simulink library "cstblocks"  (R2025b)
settings: Solver=ode45  StartTime=0.0  StopTime=10.0  RelTol=1e-3
values from neighbouring files (symbols this model uses):
  D = ltipack.lftdataFRD(IC,ltipack.LFTBlockWrapper(blk))    [ControlDesignBlock.m]    (also in DynamicBlock.m = pidstd(ltipack_ssdata(blk)); delayss.m = ltipack.ssdata(a0,b,c,[d0 q;s zeros(length(tau))],[],Ts))
  Ts = blk.Ts_    [DynamicBlock.m]    (also in delayss.m = varargin{1})
undefined symbols (not defined in the file or in its folder): AA, BB, CC, DD, Discrete, INFO, rss, set, Time, uDelay, V, xinit, yDelay
libraries: $bdroot x4, slpidlib x4, cstextras x4, sharedTrackingLibrary x3, ctrlSharedLib x1
(part 2 of 3)

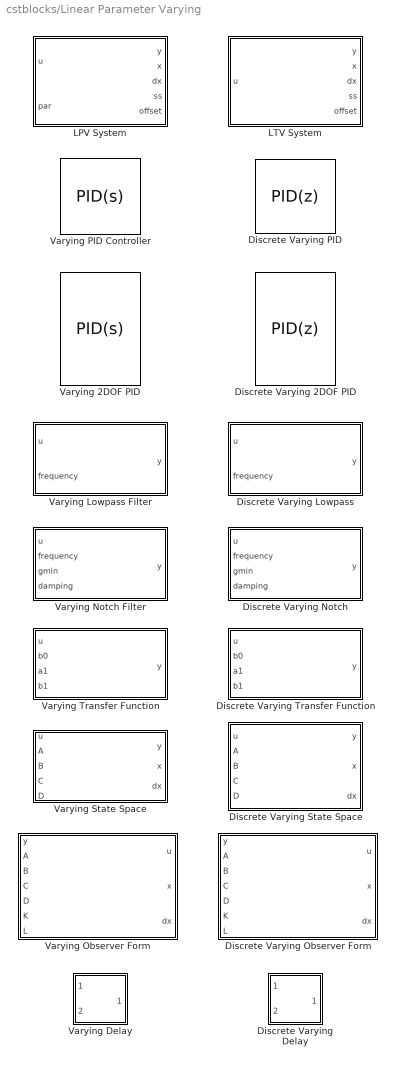
== system cstblocks/Linear Parameter Varying ==
  Discrete Varying 2DOF PID : slpidlib/PID Controller (2DOF)  Controller=PID  Form=Parallel  TimeDomain=Discrete-time  UseExternalTs=off  SampleTime=-1  IntegratorMethod=Forward Euler  FilterMethod=Forward Euler  ControllerParametersSource=external  P=1  I=1  UseKiTs=off  D=0  UseExternalDerivativeSource=off  N=100  UseFilter=on  b=1  c=1  TunerSelectOption=Transfer Function Based (PID Tuner App)  InitialConditionSource=internal  InitialConditionForIntegrator=0  InitialConditionForFilter=0  DifferentiatorICPrevScaledInput=0  ExternalReset=none  TrackingMode=off  Kt=1  LimitOutput=off  SatLimitsSource=internal  UpperSaturationLimit=inf  LowerSaturationLimit=-inf  LinearizeAsGain=on  AntiWindupMode=none  Kb=1  LimitIntegrator=off  UpperIntegratorSaturationLimit=inf  LowerIntegratorSaturationLimit=-inf  POutMin=[]  POutMax=[]  IOutMin=[]  IOutMax=[]  DOutMin=[]  DOutMax=[]  NOutMin=[]  NOutMax=[]  bOutMin=[]  bOutMax=[]  cOutMin=[]  cOutMax=[]  SumOutMin=[]  SumOutMax=[]  SaturationOutMin=[]  SaturationOutMax=[]  PParamMin=[]  PParamMax=[]  IParamMin=[]  IParamMax=[]  DParamMin=[]  DParamMax=[]  NParamMin=[]  NParamMax=[]  bParamMin=[]  bParamMax=[]  cParamMin=[]  cParamMax=[]  KbParamMin=[]  KbParamMax=[]  KtParamMin=[]  KtParamMax=[]  KbOutMin=[]  KbOutMax=[]  KtOutMin=[]  KtOutMax=[]  IntegratorOutMin=[]  IntegratorOutMax=[]  FilterOutMin=[]  FilterOutMax=[]  SumI1OutMin=[]  SumI1OutMax=[]  SumI2OutMin=[]  SumI2OutMax=[]  SumI3OutMin=[]  SumI3OutMax=[]  SumI4OutMin=[]  SumI4OutMax=[]  SumDOutMin=[]  SumDOutMax=[]  Sum1OutMin=[]  Sum1OutMax=[]  Sum2OutMin=[]  Sum2OutMax=[]  Sum3OutMin=[]  Sum3OutMax=[]  DifferentiatorOutMin=[]  DifferentiatorOutMax=[]  FilterDiffOutCoefMin=[]  FilterDiffOutCoefMax=[]  ReciprocalOutMin=[]  ReciprocalOutMax=[]  SumDenOutMin=[]  SumDenOutMax=[]  SumNumOutMin=[]  SumNumOutMax=[]  DivideOutMin=[]  DivideOutMax=[]  UdiffTsProdOutMin=[]  UdiffTsProdOutMax=[]  NTsProdOutMin=[]  NTsProdOutMax=[]  UintegralTsProdOutMin=[]  UintegralTsProdOutMax=[]  UngainTsProdOutMin=[]  UngainTsProdOutMax=[]  ClampingZeroOutDataTypeStr=Inherit: Inherit via back propagation  ClampingZeroOutMin=[]  ClampingZeroOutMax=[]  FilterDenConstantOutDataTypeStr=Inherit: Inherit via back propagation  FilterDenConstantOutMin=[]  FilterDenConstantOutMax=[]  PCopyOutDataTypeStr=Inherit: Inherit via back propagation  PCopyOutMin=[]  PCopyOutMax=[]  NCopyOutDataTypeStr=Inherit: Inherit via back propagation  NCopyOutMin=[]  NCopyOutMax=[]  IntegratorContinuousStateAttributes=''  IntegratorStateMustResolveToSignalObject=off  IntegratorRTWStateStorageClass=Auto  FilterContinuousStateAttributes=''  FilterStateMustResolveToSignalObject=off  FilterRTWStateStorageClass=Auto  ParallelPVariant=ExternalParameters  IdealPVariant=Disabled  IVariant=ExternalParameters  DVariant=ExternalParameters  bVariant=ExternalParameters  cVariant=ExternalParameters  IntegratorVariant=Discrete  SatVariant=Disabled  AWVariant=Passthrough  PCopyVariant=Disabled  TRVariant=Disabled  FdbkBlocksVariant=Forward  IdealPFdbkVariant=Disabled  SatFdbkVariant=Disabled  DerivativeFilterVariant=ForwardEulerFilter  NVariant=ExternalParameters  NCopyVariant=Disabled  FilterICVariant=InternalICsFilter  IntegratorICVariant=InternalICs  ExternalResetVariant=Disabled  TRSumVariant=Passthrough  SumFdbkVariant=Disabled  SumVariant=Sum_PID  TsampFilterVariant=InternalTs  TsampNgainVariant=Passthrough  TsampIntegralVariant=Disabled_SignalSpec  ExternalSaturationOutDataTypeStr=Inherit: Same as second input  DerivativeSourceVariant=ErrorSignal  PreIntVariant=InternalPreInt
  Discrete Varying Delay : Subsystem  mask(Discrete Varying Delay){Td=1, TdMax=10, TdFixed=[], u0=0, Ts=-1, PreventDirectFeedthrough=off}
      mask prompts: Td "Control:simulink:VaryingDelayLabel8"; TdMax "Control:simulink:VaryingDelayLabel2"; TdFixed "Control:simulink:VaryingDelayLabel4"; u0 "Control:simulink:VaryingDelayLabel5"; Ts "Control:simulink:VaryingSSLabel5"; PreventDirectFeedthrough "Control:simulink:VaryingDelayLabel9"
      mask help: Control:simulink:VaryingDelay3
      mask init:
      | df = get_param(bdroot,'dirty');
      | if ~(Ts>0 || Ts==-1)
      |    DAStudio.slerror('Control:simulink:InvalidTs',get_param(gcb,'handle'))
      | end
      | n = max([numel(Td) numel(TdMax) numel(u0)]);
      | if isscalar(Td), Td = repmat(Td,[1 n]); end
      | if isscalar(TdMax), TdMax = repmat(TdMax,[1 n]); end
      | if isscalar(u0), u0 = repmat(u0,[1 n]); end
      | if ~isequal(numel(Td),numel(TdMax),numel(u0))
      |    DAStudio.slerror('Control:simulink:VaryingDelay1',get_param(gcb,'handle'))
      | elseif any(TdFixed>n)
      |    DAStudio.slerror('Control:simulink:VaryingDelay4',get_param(gcb,'handle'))
      | end
      | 
      | % Build representation of delay vector
      | Options = struct('PreventDirectFeedthrough',PreventDirectFeedthrough);
      | controllib.internal.blocks.varying.varyingDelay(gcb,Ts,Td,TdFixed,Options);
      | set_param(bdroot,'dirty',df)
      mask Help: eval('helpview("control","DiscreteVaryingDelayBlock");')
      mask DialogControl Td Prompt: Nominal delay (number of samples):
      mask DialogControl TdMax Prompt: Maximum delay:
      mask DialogControl TdFixed Prompt: Fixed delays (indices):
      mask DialogControl u0 Prompt: Initial output:
      mask DialogControl Ts Prompt: Sample time (-1 for inherited):
      mask DialogControl PreventDirectFeedthrough Prompt: Prevent direct feedthrough with minimum delay of 1
      mask Display: block_icon('Delay')
  Discrete Varying Lowpass : Subsystem  mask(Discrete Varying Lowpass){N=1, w0=0, Ts=1}
      mask prompts: N "Control:simulink:VaryingLowpassLabel1"; w0 "Control:simulink:VaryingLowpassLabel2"; Ts "Control:simulink:VaryingLowpassLabel3"
      mask help: Control:simulink:VaryingLowpass2
      mask init:
      | if N~=round(N)
      |    hCB = get_param(gcb,'handle');
      |    DAStudio.slerror('Control:simulink:InvalidOrder',hCB)
      | elseif w0*Ts>=pi
      |    hCB = get_param(gcb,'handle');
      |    DAStudio.slerror('Control:simulink:InvalidPrewarp',hCB)
      | end
      | SimStatus = get_param(bdroot,'SimulationStatus');
      | if any(strcmp(SimStatus,{'initializing','updating','stopped'}))
      |    controllib.internal.blocks.varying.varyingLP(gcb,N,Ts)
      | end
      mask Help: eval('helpview(''control'',''VaryingLowpassDT'');')
      mask DialogControl N Prompt: Filter order:
      mask DialogControl w0 Prompt: Pre-warping frequency w0 (rad/s):
      mask DialogControl Ts Prompt: Sample time Ts:
      mask Display:
      | image('lowpass_dt.png',[0.1 0 0.8 1]);
      | port_label('input', 2, 'freq');
  Discrete Varying Notch : Subsystem  mask(Discrete Varying Notch){w0=0, Ts=1}
      mask prompts: w0 "Control:simulink:VaryingLowpassLabel2"; Ts "Control:simulink:VaryingLowpassLabel3"
      mask help: Control:simulink:VaryingNotch2
      mask init:
      | if w0*Ts>=pi
      |    hCB = get_param(gcb,'handle');
      |    DAStudio.slerror('Control:simulink:InvalidPrewarp',hCB)
      | elseif w0>0
      |    tau = tan(w0*Ts/2)/w0;
      | else
      |    tau = Ts/2;
      | end
      mask Help: eval('helpview(''control'',''VaryingNotchDT'');')
      mask DialogControl w0 Prompt: Pre-warping frequency w0 (rad/s):
      mask DialogControl Ts Prompt: Sample time Ts:
      mask Display:
      | image('notch_dt.png',[0.1 0 0.8 1])
      | port_label('input', 2, 'freq')
      | port_label('input', 3, 'gmin')
      | port_label('input', 4, 'damp')
  Discrete Varying Observer Form : Subsystem  mask(Discrete Varying Observer Form){x0=0, Ts=-1, OutputX=on, OutputDX=on}
      mask prompts: x0 "Control:simulink:VaryingSSLabel1"; Ts "Control:simulink:VaryingSSLabel5"; OutputX "Control:simulink:VaryingSSLabel3"; OutputDX "Control:simulink:VaryingSSLabel4"
      mask help: Control:simulink:VaryingObserver2
      mask init:
      | % Use exact linearization of product block
      | % pblks = find_system(gcb,'FollowLinks','on',...
      | %    'LookUnderMasks','all','SearchDepth',1,'BlockType','Product');
      | % rep = struct(...
      | %    'Specification','controllib.internal.blocks.matrixProductJacobian',...
      | %    'Type','Function',...
      | %    'ParameterNames','',...
      | %    'ParameterValues','');
      | % for i=1:numel(pblks)
      | %    set_param(pblks{i},...
      | %       'SCDEnableBlockLinearizationSpecification','on',...
      | %       'SCDBlockLinearizationSpecification',rep)
      | % end
      | SimStatus = get_param(bdroot,'SimulationStatus');
      | if any(strcmp(SimStatus,{'initializing','updating','stopped'}))
      |    controllib.internal.blocks.varying.varyingOF(gcb,OutputX,OutputDX);
      | end
      mask Help: eval('helpview(''control'',''VaryingObserverDT'');')
      mask DialogControl Ts Prompt: Sample time (-1 for inherited):
      mask DialogControl OutputX Prompt: Output states
      mask DialogControl OutputDX Prompt: Output state derivatives
      mask Display:
      | port_label('input', 1, 'y_k','texmode','on')
      | port_label('input', 2, 'A')
      | port_label('input', 3, 'B')
      | port_label('input', 4, 'C')
      | port_label('input', 5, 'D')
      | port_label('input', 6, 'K')
      | port_label('input', 7, 'L')
      | port_label('output', 1, 'u_k','texmode','on')
      | next_ = 2;
      | if OutputX
      |    port_label('output', next_, 'x_k','texmode','on')
      |    next_ = next_+1;
      | end
      | if OutputDX
      |    port_label('output', next_, 'x_{k+1}','texmode','on')
      |    next_ = next_+1;
      | end
      | text(0.5,0.7,'x_{k+1} = A x_k + B u_k + L \epsilon_k',...
      |    'horizontalAlignment', 'center','texmode','on')
      | text(0.5,0.5,'u_k = -K x_k',...
      |    'horizontalAlignment', 'center','texmode','on')
      | text(0.5,0.3,'\epsilon_k = y_k - C x_k - D u_k',...
      |    'horizontalAlignment', 'center','texmode','on')
  Discrete Varying PID : slpidlib/PID Controller  Controller=PID  Form=Parallel  TimeDomain=Discrete-time  UseExternalTs=off  SampleTime=-1  IntegratorMethod=Forward Euler  FilterMethod=Forward Euler  ControllerParametersSource=external  P=1  I=1  UseKiTs=off  D=0  UseExternalDerivativeSource=off  N=100  UseFilter=on  TunerSelectOption=Transfer Function Based (PID Tuner App)  InitialConditionSource=internal  InitialConditionForIntegrator=0  InitialConditionForFilter=0  DifferentiatorICPrevScaledInput=0  ExternalReset=none  TrackingMode=off  Kt=1  LimitOutput=off  SatLimitsSource=internal  UpperSaturationLimit=inf  LowerSaturationLimit=-inf  LinearizeAsGain=on  AntiWindupMode=none  Kb=1  LimitIntegrator=off  UpperIntegratorSaturationLimit=inf  LowerIntegratorSaturationLimit=-inf  POutMin=[]  POutMax=[]  IOutMin=[]  IOutMax=[]  DOutMin=[]  DOutMax=[]  NOutMin=[]  NOutMax=[]  SumOutMin=[]  SumOutMax=[]  SaturationOutMin=[]  SaturationOutMax=[]  PParamMin=[]  PParamMax=[]  IParamMin=[]  IParamMax=[]  DParamMin=[]  DParamMax=[]  NParamMin=[]  NParamMax=[]  KbParamMin=[]  KbParamMax=[]  KtParamMin=[]  KtParamMax=[]  KbOutMin=[]  KbOutMax=[]  KtOutMin=[]  KtOutMax=[]  IntegratorOutMin=[]  IntegratorOutMax=[]  FilterOutMin=[]  FilterOutMax=[]  SumI1OutMin=[]  SumI1OutMax=[]  SumI2OutMin=[]  SumI2OutMax=[]  SumI3OutMin=[]  SumI3OutMax=[]  SumI4OutMin=[]  SumI4OutMax=[]  SumDOutMin=[]  SumDOutMax=[]  DifferentiatorOutMin=[]  DifferentiatorOutMax=[]  FilterDiffOutCoefMin=[]  FilterDiffOutCoefMax=[]  ReciprocalOutMin=[]  ReciprocalOutMax=[]  SumDenOutMin=[]  SumDenOutMax=[]  SumNumOutMin=[]  SumNumOutMax=[]  DivideOutMin=[]  DivideOutMax=[]  UdiffTsProdOutMin=[]  UdiffTsProdOutMax=[]  NTsProdOutMin=[]  NTsProdOutMax=[]  UintegralTsProdOutMin=[]  UintegralTsProdOutMax=[]  UngainTsProdOutMin=[]  UngainTsProdOutMax=[]  ClampingZeroOutDataTypeStr=Inherit: Inherit via back propagation  ClampingZeroOutMin=[]  ClampingZeroOutMax=[]  FilterDenConstantOutDataTypeStr=Inherit: Inherit via back propagation  FilterDenConstantOutMin=[]  FilterDenConstantOutMax=[]  PCopyOutDataTypeStr=Inherit: Inherit via back propagation  PCopyOutMin=[]  PCopyOutMax=[]  NCopyOutDataTypeStr=Inherit: Inherit via back propagation  NCopyOutMin=[]  NCopyOutMax=[]  IntegratorContinuousStateAttributes=''  IntegratorStateMustResolveToSignalObject=off  IntegratorRTWStateStorageClass=Auto  FilterContinuousStateAttributes=''  FilterStateMustResolveToSignalObject=off  FilterRTWStateStorageClass=Auto  ParallelPVariant=ExternalParameters  IdealPVariant=Disabled  IVariant=ExternalParameters  DVariant=ExternalParameters  IntegratorVariant=Discrete  SatVariant=Disabled  AWVariant=Passthrough  PCopyVariant=Disabled  TRVariant=Disabled  FdbkBlocksVariant=Forward  IdealPFdbkVariant=Disabled  SatFdbkVariant=Disabled  DerivativeFilterVariant=ForwardEulerFilter  NVariant=ExternalParameters  NCopyVariant=Disabled  FilterICVariant=InternalICsFilter  IntegratorICVariant=InternalICs  ExternalResetVariant=Disabled  TRSumVariant=Passthrough  SumFdbkVariant=Disabled  SumVariant=Sum_PID  TsampFilterVariant=InternalTs  TsampNgainVariant=Passthrough  TsampIntegralVariant=Disabled_SignalSpec  ExternalSaturationOutDataTypeStr=Inherit: Same as second input  DerivativeSourceVariant=ErrorSignal  PreIntVariant=InternalPreInt
  Discrete Varying State Space : Subsystem  mask(Varying State Space){InitialConditionSource=internal, InitialCondition=0, Ts=-1, OutputX=on, OutputDX=on, Feedthrough=on, InputX0=off, InputDX0=off, InputU0=off, InputY0=off}
      mask prompts: InitialConditionSource "Simulink:blkprm_prompts:IntegratorInitCondSrc"; InitialCondition "Simulink:blkprm_prompts:IntegratorInitCond"; Ts "Control:simulink:VaryingSSLabel5"; OutputX "Control:simulink:VaryingSSLabel3"; OutputDX "Control:simulink:VaryingSSLabel4"; Feedthrough "Control:simulink:VaryingSSLabel6"; InputX0 "Control:simulink:VaryingSSLabel10"; InputDX0 "Control:simulink:VaryingSSLabel11"; InputU0 "Control:simulink:VaryingSSLabel12"; InputY0 "Control:simulink:VaryingSSLabel13"
      mask help: Control:simulink:VaryingSS1
      mask init:
      | if ~(Ts>0 || Ts==-1)
      |     DAStudio.slerror('Control:simulink:InvalidTs',get_param(gcb,'handle'))
      | end
      | if controllib.internal.blocks.safeMaskUpdate(gcb)
      |     Selection = struct('x',OutputX,'dx',OutputDX,'D',Feedthrough,...
      |         'x0',InputX0,'dx0',InputDX0,'u0',InputU0,'y0',InputY0,...
      |         'IC',strcmp(get_param(gcb,'InitialConditionSource'),'external'));
      |     if ~Selection.IC
      |         InitialCondition = InitialCondition(:);
      |     end
      |     controllib.internal.blocks.varying.varyingSS(gcb,Selection,Ts)
      | end
      mask Help: eval('helpview(''control'',''VaryingSSCT'');')
      mask TypeOptions InitialConditionSource: internal | external
      mask Callback InitialConditionSource: controllib.internal.blocks.varying.varyingSS_callback(gcb,'InitialConditionSource')
      mask DialogControl Container4 Prompt: Control:simulink:VaryingSSLabel7
      mask DialogControl InitialConditionSource Prompt: Initial condition source:
      mask DialogControl InitialCondition Prompt: Initial condition:
      mask DialogControl Ts Prompt: Sample time (-1 for inherited):
      mask DialogControl OutputX Prompt: Output states
      mask DialogControl OutputDX Prompt: Output state derivatives
      mask DialogControl Feedthrough Prompt: Enable feedthrough D
      mask DialogControl Container5 Prompt: Control:simulink:VaryingSSLabel8
      mask DialogControl InputX0 Prompt: Enable state offsets x0
      mask DialogControl InputDX0 Prompt: Enable state derivative offsets dx0
      mask DialogControl InputU0 Prompt: Enable input offsets u0
      mask DialogControl InputY0 Prompt: Enable output offsets y0
      mask Display:
      | [eqx,eqy] = controllib.internal.blocks.varying.varyingSS_icon(false,Feedthrough,InputX0,InputDX0,InputU0,InputY0);
      | text(0.5,0.65,eqx,'horizontalAlignment', 'center','texmode','on')
      | text(0.5,0.35,eqy,'horizontalAlignment', 'center','texmode','on')
      | port_label('input', 1, 'u_k','texmode','on')
      | port_label('input', 2, 'A')
      | port_label('input', 3, 'B')
      | port_label('input', 4, 'C')
      | port_label('output', 1, 'y_k','texmode','on')
      | nout = 1;
      | if OutputX
      |    nout = nout+1;
      |    port_label('output', nout, 'x_k','texmode','on')
      | end
      | if OutputDX
      |    nout = nout+1;
      |    port_label('output', nout, 'x_{k+1}','texmode','on')
      | end
      | nin = 4;
      | if Feedthrough
      |    nin = nin+1;
      |    port_label('input', nin, 'D')
      | end
      | if InputDX0
      |    nin = nin+1;
      |    port_label('input', nin, 'dx0')
      | end
      | if InputX0
      |    nin = nin+1;
      |    port_label('input', nin, 'x0')
      | end
      | if InputU0
      |    nin = nin+1;
      |    port_label('input', nin, 'u0')
      | end
      | if InputY0
      |    nin = nin+1;
      |    port_label('input', nin, 'y0')
      | end
      | if strcmp(get_param(gcb,'InitialConditionSource'),'external')
      |    nin = nin+1;
      |    port_label('input', nin, 'IC')
      | end
  Discrete Varying Transfer Function : Subsystem  mask(Discrete Varying Transfer Function){N=1, Feedthrough=on, Ts=-1}
      mask prompts: N "Control:simulink:VaryingTFLabel1"; Feedthrough "Control:simulink:VaryingSSLabel6"; Ts "Control:simulink:VaryingTFLabel2"
      mask help: Control:simulink:VaryingTF2
      mask init:
      | if N~=round(N)
      |    hCB = get_param(gcb,'handle');
      |    DAStudio.slerror('Control:simulink:InvalidOrder',hCB)
      | elseif ~(Ts>0 || Ts==-1)
      |    hCB = get_param(gcb,'handle');
      |    DAStudio.slerror('Control:simulink:InvalidTs',hCB)   
      | end
      | SimStatus = get_param(bdroot,'SimulationStatus');
      | if any(strcmp(SimStatus,{'initializing','updating','stopped'}))
      |    controllib.internal.blocks.varying.varyingTF(gcb,N,Ts,Feedthrough)
      | end
      mask Help: eval('helpview(''control'',''VaryingTFDT'');')
      mask DialogControl N Prompt: Transfer function order:
      mask DialogControl Feedthrough Prompt: Enable feedthrough D
      mask DialogControl Ts Prompt: Sample time (-1 for inherited):
      mask Display:
      | port_label('input',3,'a1');
      | port_label('input',2,'b0');
      | port_label('input',4,'b1');
      | plot([0.325 0.675],[0.5 0.5])
      | text(0.5, 0.7, 'b_0 + b_1 z^{-1}' ,...
      |         'horizontalAlignment', 'center','texmode','on')
      | text(0.5, 0.3, '1 + a_1 z^{-1}' ,...
      |         'horizontalAlignment', 'center','texmode','on')
  LPV System : Subsystem  mask(LPV Block){sys=set(rss(1,1,1,3),'SamplingGrid',struct('p',[1 2 3])), InitialConditionSource=internal, InitialCondition=0, opSpecOption=Specify offsets as double arrays, uOffset=0, yOffset=0, xOffset=0, opEquilOption=on, dxOffset=0, Offset=struct, AFixed=false, BFixed=false, CFixed=false, DFixed=false, uDelayFixed=false, yDelayFixed=false, iDelayFixed=false, sysFixedOption=First model in state-space array, sysFixed=[], IMethod=Linear, EMethod=Clip, IndexSearch=Binary search, IndexBegin=on, OutputX=on, OutputXdot=on, OutputLTI=on, OutputOP=on, DataType=double, InitBufferSize=1024, FixedBuffer=off, SimMode=Interpreted execution}
      mask prompts: sys "Control:simulink:LPVMask14"; InitialConditionSource "Simulink:blkprm_prompts:IntegratorInitCondSrc"; InitialCondition "Simulink:blkprm_prompts:IntegratorInitCond"; uOffset "Control:simulink:LPVMask8"; yOffset "Control:simulink:LPVMask9"; xOffset "Control:simulink:LPVMask10"; opEquilOption "Control:simulink:LPVMask11b"; dxOffset "Control:simulink:LPVMask11c"; Offset "Control:simulink:LPVMask48"; AFixed "Control:simulink:LPVMask31"; BFixed "Control:simulink:LPVMask32"; CFixed "Control:simulink:LPVMask33"; DFixed "Control:simulink:LPVMask34"; uDelayFixed "Control:simulink:LPVMask35"; yDelayFixed "Control:simulink:LPVMask36"; iDelayFixed "Control:simulink:LPVMask37"; sysFixed "Control:simulink:LPVMask18"; IMethod "Control:simulink:LPVMask23"; EMethod "Control:simulink:LPVMask24"; IndexSearch "Control:simulink:LPVMask25"; IndexBegin "Control:simulink:LPVMask26"; OutputX "Control:simulink:LPVMask27"; OutputXdot "Control:simulink:LPVMask28"; OutputLTI "Control:simulink:LPVMask29"; OutputOP "Control:simulink:LPVMask30"; DataType "Control:simulink:LPVMask40"; InitBufferSize "Control:simulink:LPVMask42"; FixedBuffer "Control:simulink:LPVMask44"; SimMode "Control:simulink:LPVMask41"
      mask help: Control:simulink:LPVMask1
      mask init:
      | % if isequal(sys,[])
      | %     return
      | % end
      | model = bdroot;
      | df = get_param(model,'dirty');
      | 
      | % Configure ports
      | InputIC =  strcmp(get_param(gcb,'InitialConditionSource'),'external');
      | controllib.internal.blocks.lpv.configurePorts(gcb,...
      |     InputIC,OutputX,OutputXdot,OutputLTI,OutputOP);
      | 
      | % Process data
      | Fixed = struct('A',AFixed,'B',BFixed,'C',CFixed,'D',DFixed,...
      |     'uDelay',uDelayFixed,'yDelay',yDelayFixed,'xDelay',iDelayFixed);
      | if sysFixedOption==1
      |     sysNominal = [];
      | else
      |     sysNominal = sysFixed;
      | end
      | try
      |     %fprintf('opSpecOption=%d\n',opSpecOption)
      |     switch opSpecOption
      |         case 1
      |             OffsetData = struct('dx',dxOffset,'x',xOffset,'u',uOffset,...
      |                 'y',yOffset,'EQUIL',opEquilOption);
      |         case 2
      |             OffsetData = Offset;
      |         case 3
      |             OffsetData = [];
      |     end
      |     [V,INFO,InitialCondition,Ts] = controllib.internal.blocks.lpv.lpvmaskData(...
      |         gcb,sys,InitialCondition,OffsetData,sysNominal,...
      |         Fixed,IMethod,EMethod,DataType,opSpecOption);
      | catch ME
      |     throwAsCaller(MSLException(get_param(gcb,'handle'),ME.identifier,ME.message))
      | end
      | 
      | % Update contents
      | controllib.internal.blocks.lpv.lpvmaskUpdate(gcb,INFO,Ts,...
      |     InputIC, OutputX, OutputXdot, OutputLTI, OutputOP, ...
      |     IndexSearch,IndexBegin,InitBufferSize,FixedBuffer);
      | try
      |     % Attempt to modify locked library -> error
      |     set_param(model,'dirty',df)
      | end
      mask Help: eval('helpview("control","LPVSystemBlock");')
      mask Callback sys: controllib.internal.blocks.lpv.lpvmaskCallback(gcb,'SystemArray')
      mask TypeOptions InitialConditionSource: internal | external
      mask Callback InitialConditionSource: controllib.internal.blocks.lpv.lpvmaskCallback(gcb,'InitialConditionSource')
      mask TypeOptions opSpecOption: Control:simulink:LPVMask45 | Control:simulink:LPVMask46 | Control:simulink:LPVMask47
      mask Callback opSpecOption: controllib.internal.blocks.lpv.lpvmaskCallback(gcb,'OPSpecOption')
      mask Callback opEquilOption: controllib.internal.blocks.lpv.lpvmaskCallback(gcb,'OPEquilOption')
      mask TypeOptions sysFixedOption: Control:simulink:LPVMask16b | Control:simulink:LPVMask17b
      mask Callback sysFixedOption: controllib.internal.blocks.lpv.lpvmaskCallback(gcb,'SysFixedOption')
      mask TypeOptions IMethod: Flat | Nearest | Linear
      mask TypeOptions EMethod: Clip | Linear
      mask TypeOptions IndexSearch: Binary search | Linear search
      mask TypeOptions DataType: double | single
      mask TypeOptions SimMode: Interpreted execution | Code generation
      mask DialogControl Container4 Prompt: Control:simulink:LPVMask2
      mask DialogControl Container5 Prompt: Control:simulink:LPVMask6
      mask DialogControl sys Prompt: State-space array:
      mask DialogControl InitialConditionSource Prompt: Initial condition source:
      mask DialogControl InitialCondition Prompt: Initial condition:
      mask DialogControl Container6 Prompt: Control:simulink:LPVMask7
      mask DialogControl uOffset Prompt: Input offset:
      mask DialogControl yOffset Prompt: Output offset:
      mask DialogControl xOffset Prompt: State offset:
      mask DialogControl Control5 Prompt: Control:simulink:LPVMask11a
      mask DialogControl opEquilOption Prompt: Assume equilibrium operating conditions
      mask DialogControl dxOffset Prompt: Offset value:
      mask DialogControl Offset Prompt: Struct array:
      mask DialogControl Container7 Prompt: Control:simulink:LPVMask5
      mask DialogControl Control2 Prompt: Control:simulink:LPVMask12
      mask DialogControl Container10 Prompt: Control:simulink:LPVMask19
      mask DialogControl Control4 Prompt: Control:simulink:LPVMask22
      mask DialogControl AFixed Prompt: A matrix:
      mask DialogControl BFixed Prompt: B matrix:
      mask DialogControl CFixed Prompt: C matrix:
      mask DialogControl DFixed Prompt: D matrix:
      mask DialogControl uDelayFixed Prompt: Input delay:
      mask DialogControl yDelayFixed Prompt: Output delay:
      mask DialogControl iDelayFixed Prompt: Internal delay:
      mask DialogControl Container9 Prompt: Control:simulink:LPVMask15
      mask DialogControl Control7 Prompt: Control:simulink:LPVMask15b
      mask DialogControl sysFixed Prompt: Custom model:
      mask DialogControl Container13 Prompt: Control:simulink:LPVMask3
      mask DialogControl IMethod Prompt: Interpolation method:
      mask DialogControl EMethod Prompt: Extrapolation method:
      mask DialogControl IndexSearch Prompt: Index search method:
      mask DialogControl IndexBegin Prompt: Begin index search using previous index result
      mask DialogControl Container14 Prompt: Control:simulink:LPVMask4
      mask DialogControl Container15 Prompt: Control:simulink:LPVMask38
      mask DialogControl OutputX Prompt: Output states
      mask DialogControl OutputXdot Prompt: Output state derivatives (continuous-time) or updates (discrete-time)
      mask DialogControl OutputLTI Prompt: Output interpolated state-space data
      mask DialogControl OutputOP Prompt: Output interpolated offsets
      mask DialogControl Container17 Prompt: Control:simulink:LPVMask39
      mask DialogControl DataType Prompt: Block data type (discrete-time case only):
      mask DialogControl InitBufferSize Prompt: Initial buffer size for delays:
      mask DialogControl FixedBuffer Prompt: Use fixed buffer size
      mask DialogControl SimMode Prompt: Simulation mode for MATLAB System blocks:
      mask Display:
      | fprintf('LPV')
      | port_label('input', 1, 'u')
      | port_label('input', 2, 'par')
      | port_label('output', 1, 'y')
      | next_ = 2;
      | 
      | if OutputX
      |    port_label('output', next_, 'x')
      |    next_ = next_+1;
      | end
      | 
      | if OutputXdot
      |    port_label('output', next_, 'dx')
      |    next_ = next_+1;
      | end
      | 
      | if OutputLTI
      |    port_label('output', next_, 'ss')
      |    next_ = next_+1;
      | end
      | 
      | if OutputOP
      |    port_label('output', next_, 'offset')
      | end
      | 
      | if InputIC
      |    port_label('input', 3, 'IC')
      | end
  LTV System : Subsystem  mask(LTV Block){sys=set(rss(1,1,1,3),'SamplingGrid',struct('Time',[0 1 2])), InitialConditionSource=internal, InitialCondition=0, opSpecOption=Specify offsets as double arrays, uOffset=0, yOffset=0, xOffset=0, opEquilOption=on, dxOffset=0, Offset=struct, AFixed=false, BFixed=false, CFixed=false, DFixed=false, uDelayFixed=false, yDelayFixed=false, iDelayFixed=false, sysFixedOption=First model in state-space array, sysFixed=[], IMethod=Linear, EMethod=Clip, IndexSearch=Binary search, IndexBegin=on, OutputX=on, OutputXdot=on, OutputLTI=on, OutputOP=on, DataType=double, SimMode=Interpreted execution, InitBufferSize=1024, FixedBuffer=off}
      mask prompts: sys "Control:simulink:LPVMask14"; InitialConditionSource "Simulink:blkprm_prompts:IntegratorInitCondSrc"; InitialCondition "Simulink:blkprm_prompts:IntegratorInitCond"; uOffset "Control:simulink:LPVMask8"; yOffset "Control:simulink:LPVMask9"; xOffset "Control:simulink:LPVMask10"; opEquilOption "Control:simulink:LPVMask11b"; dxOffset "Control:simulink:LPVMask11c"; Offset "Control:simulink:LPVMask48"; AFixed "Control:simulink:LPVMask31"; BFixed "Control:simulink:LPVMask32"; CFixed "Control:simulink:LPVMask33"; DFixed "Control:simulink:LPVMask34"; uDelayFixed "Control:simulink:LPVMask35"; yDelayFixed "Control:simulink:LPVMask36"; iDelayFixed "Control:simulink:LPVMask37"; sysFixed "Control:simulink:LPVMask18"; IMethod "Control:simulink:LPVMask23"; EMethod "Control:simulink:LPVMask24"; IndexSearch "Control:simulink:LPVMask25"; IndexBegin "Control:simulink:LPVMask26"; OutputX "Control:simulink:LPVMask27"; OutputXdot "Control:simulink:LPVMask28"; OutputLTI "Control:simulink:LPVMask29"; OutputOP "Control:simulink:LPVMask30"; DataType "Control:simulink:LPVMask40"; SimMode "Control:simulink:LPVMask41"; InitBufferSize "Control:simulink:LPVMask42"; FixedBuffer "Control:simulink:LPVMask44"
      mask help: Control:simulink:LTVMask1
      mask init:
      | % if isequal(sys,[])
      | %     return
      | % end
      | model = bdroot;
      | df = get_param(model,'dirty');
      | 
      | % Configure ports
      | InputIC =  strcmp(get_param(gcb,'InitialConditionSource'),'external');
      | controllib.internal.blocks.lpv.configurePorts(gcb,...
      |     InputIC,OutputX,OutputXdot,OutputLTI,OutputOP);
      | 
      | % Process data
      | Fixed = struct('A',AFixed,'B',BFixed,'C',CFixed,'D',DFixed,...
      |     'uDelay',uDelayFixed,'yDelay',yDelayFixed,'xDelay',iDelayFixed);
      | if sysFixedOption==1
      |     sysNominal = [];
      | else
      |     sysNominal = sysFixed;
      | end
      | try
      |     switch opSpecOption
      |         case 1
      |             OffsetData = struct('dx',dxOffset,'x',xOffset,'u',uOffset,'y',yOffset,...
      |                 'EQUIL',opEquilOption);
      |         case 2
      |             OffsetData = Offset;
      |         case 3
      |             OffsetData = [];
      |     end
      |     [V,INFO,InitialCondition,Ts] = controllib.internal.blocks.lpv.ltvmaskData(...
      |         gcb,sys,InitialCondition,OffsetData,sysNominal,...
      |         Fixed,IMethod,EMethod,DataType,opSpecOption);
      | catch ME
      |     throwAsCaller(MSLException(get_param(gcb,'handle'),ME.identifier,ME.message))
      | end
      | 
      | % Update contents
      | controllib.internal.blocks.lpv.lpvmaskUpdate(gcb,INFO,Ts,...
      |     InputIC, OutputX, OutputXdot, OutputLTI, OutputOP, ...
      |     IndexSearch,IndexBegin,InitBufferSize,FixedBuffer);
      | try
      |     % Attempt to modify locked library -> error
      |     set_param(model,'dirty',df)
      | end
      mask Help: eval('helpview("control","LTVSystemBlock");')
      mask Callback sys: controllib.internal.blocks.lpv.lpvmaskCallback(gcb,'SystemArray')
      mask TypeOptions InitialConditionSource: internal | external
      mask Callback InitialConditionSource: controllib.internal.blocks.lpv.lpvmaskCallback(gcb,'InitialConditionSource')
      mask TypeOptions opSpecOption: Control:simulink:LPVMask45 | Control:simulink:LPVMask46 | Control:simulink:LPVMask47
      mask Callback opSpecOption: controllib.internal.blocks.lpv.lpvmaskCallback(gcb,'OPSpecOption')
      mask Callback opEquilOption: controllib.internal.blocks.lpv.lpvmaskCallback(gcb,'OPEquilOption')
      mask TypeOptions sysFixedOption: Control:simulink:LPVMask16b | Control:simulink:LPVMask17b
      mask Callback sysFixedOption: controllib.internal.blocks.lpv.lpvmaskCallback(gcb,'SysFixedOption')
      mask TypeOptions IMethod: Flat | Nearest | Linear
      mask TypeOptions EMethod: Clip | Linear
      mask TypeOptions IndexSearch: Binary search | Linear search
      mask TypeOptions DataType: double | single
      mask TypeOptions SimMode: Interpreted execution | Code generation
      mask DialogControl Container4 Prompt: Control:simulink:LTVMask2
      mask DialogControl Container5 Prompt: Control:simulink:LPVMask6
      mask DialogControl sys Prompt: State-space array:
      mask DialogControl InitialConditionSource Prompt: Initial condition source:
      mask DialogControl InitialCondition Prompt: Initial condition:
      mask DialogControl Container6 Prompt: Control:simulink:LPVMask7
      mask DialogControl uOffset Prompt: Input offset:
      mask DialogControl yOffset Prompt: Output offset:
      mask DialogControl xOffset Prompt: State offset:
      mask DialogControl Control5 Prompt: Control:simulink:LPVMask11a
      mask DialogControl opEquilOption Prompt: Assume equilibrium operating conditions
      mask DialogControl dxOffset Prompt: Offset value:
      mask DialogControl Offset Prompt: Struct array:
      mask DialogControl Container7 Prompt: Control:simulink:LPVMask5
      mask DialogControl Control2 Prompt: Control:simulink:LTVMask3
      mask DialogControl Container10 Prompt: Control:simulink:LPVMask19
      mask DialogControl Control4 Prompt: Control:simulink:LPVMask22
      mask DialogControl AFixed Prompt: A matrix:
      mask DialogControl BFixed Prompt: B matrix:
      mask DialogControl CFixed Prompt: C matrix:
      mask DialogControl DFixed Prompt: D matrix:
      mask DialogControl uDelayFixed Prompt: Input delay:
      mask DialogControl yDelayFixed Prompt: Output delay:
      mask DialogControl iDelayFixed Prompt: Internal delay:
      mask DialogControl Container9 Prompt: Control:simulink:LPVMask15
      mask DialogControl Control7 Prompt: Control:simulink:LPVMask15b
      mask DialogControl sysFixed Prompt: Custom model:
      mask DialogControl Container13 Prompt: Control:simulink:LPVMask3
      mask DialogControl IMethod Prompt: Interpolation method:
      mask DialogControl EMethod Prompt: Extrapolation method:
      mask DialogControl IndexSearch Prompt: Index search method:
      mask DialogControl IndexBegin Prompt: Begin index search using previous index result
      mask DialogControl Container14 Prompt: Control:simulink:LPVMask4
      mask DialogControl Container15 Prompt: Control:simulink:LPVMask38
      mask DialogControl OutputX Prompt: Output states
      mask DialogControl OutputXdot Prompt: Output state derivatives (continuous-time) or updates (discrete-time)
      mask DialogControl OutputLTI Prompt: Output interpolated state-space data
      mask DialogControl OutputOP Prompt: Output interpolated offsets
      mask DialogControl Container17 Prompt: Control:simulink:LPVMask39
      mask DialogControl DataType Prompt: Block data type (discrete-time case only):
      mask DialogControl SimMode Prompt: Simulation mode for MATLAB System blocks:
      mask DialogControl InitBufferSize Prompt: Initial buffer size for delays:
      mask DialogControl FixedBuffer Prompt: Use fixed buffer size
      mask Display:
      | fprintf('LTV')
      | port_label('input', 1, 'u')
      | port_label('output', 1, 'y')
      | next_ = 2;
      | 
      | if OutputX
      |    port_label('output', next_, 'x')
      |    next_ = next_+1;
      | end
      | 
      | if OutputXdot
      |    port_label('output', next_, 'dx')
      |    next_ = next_+1;
      | end
      | 
      | if OutputLTI
      |    port_label('output', next_, 'ss')
      |    next_ = next_+1;
      | end
      | 
      | if OutputOP
      |    port_label('output', next_, 'offset')
      | end
      | 
      | if InputIC
      |    port_label('input', 2, 'IC')
      | end
  Varying 2DOF PID : slpidlib/PID Controller (2DOF)  Controller=PID  Form=Parallel  TimeDomain=Continuous-time  UseExternalTs=off  SampleTime=-1  IntegratorMethod=Forward Euler  FilterMethod=Forward Euler  ControllerParametersSource=external  P=1  I=1  UseKiTs=off  D=0  UseExternalDerivativeSource=off  N=100  UseFilter=on  b=1  c=1  TunerSelectOption=Transfer Function Based (PID Tuner App)  InitialConditionSource=internal  InitialConditionForIntegrator=0  InitialConditionForFilter=0  DifferentiatorICPrevScaledInput=0  ExternalReset=none  TrackingMode=off  Kt=1  LimitOutput=off  SatLimitsSource=internal  UpperSaturationLimit=inf  LowerSaturationLimit=-inf  LinearizeAsGain=on  AntiWindupMode=none  Kb=1  LimitIntegrator=off  UpperIntegratorSaturationLimit=inf  LowerIntegratorSaturationLimit=-inf  POutMin=[]  POutMax=[]  IOutMin=[]  IOutMax=[]  DOutMin=[]  DOutMax=[]  NOutMin=[]  NOutMax=[]  bOutMin=[]  bOutMax=[]  cOutMin=[]  cOutMax=[]  SumOutMin=[]  SumOutMax=[]  SaturationOutMin=[]  SaturationOutMax=[]  PParamMin=[]  PParamMax=[]  IParamMin=[]  IParamMax=[]  DParamMin=[]  DParamMax=[]  NParamMin=[]  NParamMax=[]  bParamMin=[]  bParamMax=[]  cParamMin=[]  cParamMax=[]  KbParamMin=[]  KbParamMax=[]  KtParamMin=[]  KtParamMax=[]  KbOutMin=[]  KbOutMax=[]  KtOutMin=[]  KtOutMax=[]  IntegratorOutMin=[]  IntegratorOutMax=[]  FilterOutMin=[]  FilterOutMax=[]  SumI1OutMin=[]  SumI1OutMax=[]  SumI2OutMin=[]  SumI2OutMax=[]  SumI3OutMin=[]  SumI3OutMax=[]  SumI4OutMin=[]  SumI4OutMax=[]  SumDOutMin=[]  SumDOutMax=[]  Sum1OutMin=[]  Sum1OutMax=[]  Sum2OutMin=[]  Sum2OutMax=[]  Sum3OutMin=[]  Sum3OutMax=[]  DifferentiatorOutMin=[]  DifferentiatorOutMax=[]  FilterDiffOutCoefMin=[]  FilterDiffOutCoefMax=[]  ReciprocalOutMin=[]  ReciprocalOutMax=[]  SumDenOutMin=[]  SumDenOutMax=[]  SumNumOutMin=[]  SumNumOutMax=[]  DivideOutMin=[]  DivideOutMax=[]  UdiffTsProdOutMin=[]  UdiffTsProdOutMax=[]  NTsProdOutMin=[]  NTsProdOutMax=[]  UintegralTsProdOutMin=[]  UintegralTsProdOutMax=[]  UngainTsProdOutMin=[]  UngainTsProdOutMax=[]  ClampingZeroOutDataTypeStr=Inherit: Inherit via back propagation  ClampingZeroOutMin=[]  ClampingZeroOutMax=[]  FilterDenConstantOutDataTypeStr=Inherit: Inherit via back propagation  FilterDenConstantOutMin=[]  FilterDenConstantOutMax=[]  PCopyOutDataTypeStr=Inherit: Inherit via back propagation  PCopyOutMin=[]  PCopyOutMax=[]  NCopyOutDataTypeStr=Inherit: Inherit via back propagation  NCopyOutMin=[]  NCopyOutMax=[]  IntegratorContinuousStateAttributes=''  IntegratorStateMustResolveToSignalObject=off  IntegratorRTWStateStorageClass=Auto  FilterContinuousStateAttributes=''  FilterStateMustResolveToSignalObject=off  FilterRTWStateStorageClass=Auto  ParallelPVariant=ExternalParameters  IdealPVariant=Disabled  IVariant=ExternalParameters  DVariant=ExternalParameters  bVariant=ExternalParameters  cVariant=ExternalParameters  IntegratorVariant=Continuous  SatVariant=Disabled  AWVariant=Passthrough  PCopyVariant=Disabled  TRVariant=Disabled  FdbkBlocksVariant=Forward  IdealPFdbkVariant=Disabled  SatFdbkVariant=Disabled  DerivativeFilterVariant=ContFilter  NVariant=ExternalParameters  NCopyVariant=Disabled  FilterICVariant=InternalICsFilter  IntegratorICVariant=InternalICs  ExternalResetVariant=Disabled  TRSumVariant=Passthrough  SumFdbkVariant=Disabled  SumVariant=Sum_PID  TsampFilterVariant=InternalTs  TsampNgainVariant=Passthrough  TsampIntegralVariant=Disabled_SignalSpec  ExternalSaturationOutDataTypeStr=Inherit: Same as second input  DerivativeSourceVariant=ErrorSignal  PreIntVariant=InternalPreInt
  Varying Delay : Subsystem  mask(Varying Delay){Td=1, TdMax=10, TdMin=0, TdFixed=[], u0=0, bufsize=1024, FixedBuffer=off, PadeOrder=0}
      mask prompts: Td "Control:simulink:VaryingDelayLabel1"; TdMax "Control:simulink:VaryingDelayLabel2"; TdMin "Control:simulink:VaryingDelayLabel3"; TdFixed "Control:simulink:VaryingDelayLabel4"; u0 "Control:simulink:VaryingDelayLabel5"; bufsize "Control:simulink:VaryingDelayLabel6"; FixedBuffer "Control:simulink:VaryingDelayLabel7"; PadeOrder "Simulink:blkprm_prompts:TransDelayPadeOrder"
      mask help: Control:simulink:VaryingDelay2
      mask init:
      | df = get_param(bdroot,'dirty');
      | n = max([numel(Td) numel(TdMax) numel(u0) numel(PadeOrder)]);
      | if isscalar(Td), Td = repmat(Td,[1 n]); end
      | if isscalar(TdMax), TdMax = repmat(TdMax,[1 n]); end
      | if isscalar(u0), u0 = repmat(u0,[1 n]); end
      | if isscalar(PadeOrder), PadeOrder = repmat(PadeOrder,[1 n]); end
      | if ~isequal(numel(Td),numel(TdMax),numel(u0),numel(PadeOrder))
      |    DAStudio.slerror('Control:simulink:VaryingDelay1',get_param(gcb,'handle'))
      | elseif any(TdFixed>n)
      |    DAStudio.slerror('Control:simulink:VaryingDelay4',get_param(gcb,'handle'))
      | end
      | 
      | % Build representation of delay vector
      | if TdMin>0
      |     ZeroDelay = 'off';
      | else
      |     ZeroDelay = 'on';
      | end
      | Options = struct('ZeroDelay',ZeroDelay,'FixedBuffer',FixedBuffer);
      | controllib.internal.blocks.varying.varyingDelay(gcb, 0, Td, TdFixed, Options);
      | set_param(bdroot,'dirty',df)
      mask Help: eval('helpview("control","VaryingDelayBlock");')
      mask DialogControl Td Prompt: Nominal delay:
      mask DialogControl TdMax Prompt: Maximum delay:
      mask DialogControl TdMin Prompt: Minimum delay:
      mask DialogControl TdFixed Prompt: Fixed delays (indices):
      mask DialogControl u0 Prompt: Initial output:
      mask DialogControl bufsize Prompt: Initial buffer size:
      mask DialogControl FixedBuffer Prompt: Use fixed buffer size
      mask DialogControl PadeOrder Prompt: Pade order (for linearization):
      mask Display: block_icon('Delay')
  Varying Lowpass Filter : Subsystem  mask(Varying Lowpass Filter){N=1}
      mask prompts: N "Control:simulink:VaryingLowpassLabel1"
      mask help: Control:simulink:VaryingLowpass1
      mask init:
      | if N~=round(N)
      |    hCB = get_param(gcb,'handle');
      |    DAStudio.slerror('Control:simulink:InvalidOrder',hCB)
      | end
      | SimStatus = get_param(bdroot,'SimulationStatus');
      | if any(strcmp(SimStatus,{'initializing','updating','stopped'}))
      |    controllib.internal.blocks.varying.varyingLP(gcb,N,0)
      | end
      mask Help: eval('helpview(''control'',''VaryingLowpassCT'');')
      mask DialogControl N Prompt: Filter order:
      mask Display:
      | image('lowpass_ct.png',[0.1 0 0.8 1]);
      | port_label('input', 2, 'freq');
  Varying Notch Filter : Subsystem  mask(Varying Notch Filter){}
      mask help: Control:simulink:VaryingNotch1
      mask Help: eval('helpview(''control'',''VaryingNotchCT'');')
      mask Display:
      | image('notch_ct.png',[0.1 0 0.8 1])
      | port_label('input', 2, 'freq')
      | port_label('input', 3, 'gmin')
      | port_label('input', 4, 'damp')
  Varying Observer Form : Subsystem  mask(Varying Observer Form){x0=0, xNames='', OutputX=on, OutputDX=on}
      mask prompts: x0 "Control:simulink:VaryingSSLabel1"; xNames "Control:simulink:VaryingSSLabel2"; OutputX "Control:simulink:VaryingSSLabel3"; OutputDX "Control:simulink:VaryingSSLabel4"
      mask help: Control:simulink:VaryingObserver1
      mask init:
      | % Use exact linearization of product block
      | % pblks = find_system(gcb,'FollowLinks','on',...
      | %    'LookUnderMasks','all','SearchDepth',1,'BlockType','Product');
      | % rep = struct(...
      | %    'Specification','controllib.internal.blocks.matrixProductJacobian',...
      | %    'Type','Function',...
      | %    'ParameterNames','',...
      | %    'ParameterValues','');
      | % for i=1:numel(pblks)
      | %    set_param(pblks{i},...
      | %       'SCDEnableBlockLinearizationSpecification','on',...
      | %       'SCDBlockLinearizationSpecification',rep)
      | % end
      | SimStatus = get_param(bdroot,'SimulationStatus');
      | if any(strcmp(SimStatus,{'initializing','updating','stopped'}))
      |    controllib.internal.blocks.varying.varyingOF(gcb,OutputX,OutputDX);
      | end
      mask Help: eval('helpview(''control'',''VaryingObserverCT'');')
      mask DialogControl xNames Prompt: State names (e.g., 'position'):
      mask DialogControl OutputX Prompt: Output states
      mask DialogControl OutputDX Prompt: Output state derivatives
      mask Display:
      | port_label('input', 1, 'y')
      | port_label('input', 2, 'A')
      | port_label('input', 3, 'B')
      | port_label('input', 4, 'C')
      | port_label('input', 5, 'D')
      | port_label('input', 6, 'K')
      | port_label('input', 7, 'L')
      | port_label('output', 1, 'u')
      | next_ = 2;
      | if OutputX
      |    port_label('output', next_, 'x_e','texmode','on')
      |    next_ = next_+1;
      | end
      | if OutputDX
      |    port_label('output', next_, 'dx_e','texmode','on')
      |    next_ = next_+1;
      | end
      | text(0.5,0.7,'dx_e = A x_e + B u + L \epsilon',...
      |    'horizontalAlignment', 'center','texmode','on')
      | text(0.5,0.5,'u = -K x_e',...
      |    'horizontalAlignment', 'center','texmode','on')
      | text(0.5,0.3,'\epsilon = y - C x_e - D u',...
      |    'horizontalAlignment', 'center','texmode','on')
  Varying PID Controller : slpidlib/PID Controller  Controller=PID  Form=Parallel  TimeDomain=Continuous-time  UseExternalTs=off  SampleTime=-1  IntegratorMethod=Forward Euler  FilterMethod=Forward Euler  ControllerParametersSource=external  P=1  I=1  UseKiTs=off  D=0  UseExternalDerivativeSource=off  N=100  UseFilter=on  TunerSelectOption=Transfer Function Based (PID Tuner App)  InitialConditionSource=internal  InitialConditionForIntegrator=0  InitialConditionForFilter=0  DifferentiatorICPrevScaledInput=0  ExternalReset=none  TrackingMode=off  Kt=1  LimitOutput=off  SatLimitsSource=internal  UpperSaturationLimit=inf  LowerSaturationLimit=-inf  LinearizeAsGain=on  AntiWindupMode=none  Kb=1  LimitIntegrator=off  UpperIntegratorSaturationLimit=inf  LowerIntegratorSaturationLimit=-inf  POutMin=[]  POutMax=[]  IOutMin=[]  IOutMax=[]  DOutMin=[]  DOutMax=[]  NOutMin=[]  NOutMax=[]  SumOutMin=[]  SumOutMax=[]  SaturationOutMin=[]  SaturationOutMax=[]  PParamMin=[]  PParamMax=[]  IParamMin=[]  IParamMax=[]  DParamMin=[]  DParamMax=[]  NParamMin=[]  NParamMax=[]  KbParamMin=[]  KbParamMax=[]  KtParamMin=[]  KtParamMax=[]  KbOutMin=[]  KbOutMax=[]  KtOutMin=[]  KtOutMax=[]  IntegratorOutMin=[]  IntegratorOutMax=[]  FilterOutMin=[]  FilterOutMax=[]  SumI1OutMin=[]  SumI1OutMax=[]  SumI2OutMin=[]  SumI2OutMax=[]  SumI3OutMin=[]  SumI3OutMax=[]  SumI4OutMin=[]  SumI4OutMax=[]  SumDOutMin=[]  SumDOutMax=[]  DifferentiatorOutMin=[]  DifferentiatorOutMax=[]  FilterDiffOutCoefMin=[]  FilterDiffOutCoefMax=[]  ReciprocalOutMin=[]  ReciprocalOutMax=[]  SumDenOutMin=[]  SumDenOutMax=[]  SumNumOutMin=[]  SumNumOutMax=[]  DivideOutMin=[]  DivideOutMax=[]  UdiffTsProdOutMin=[]  UdiffTsProdOutMax=[]  NTsProdOutMin=[]  NTsProdOutMax=[]  UintegralTsProdOutMin=[]  UintegralTsProdOutMax=[]  UngainTsProdOutMin=[]  UngainTsProdOutMax=[]  ClampingZeroOutDataTypeStr=Inherit: Inherit via back propagation  ClampingZeroOutMin=[]  ClampingZeroOutMax=[]  FilterDenConstantOutDataTypeStr=Inherit: Inherit via back propagation  FilterDenConstantOutMin=[]  FilterDenConstantOutMax=[]  PCopyOutDataTypeStr=Inherit: Inherit via back propagation  PCopyOutMin=[]  PCopyOutMax=[]  NCopyOutDataTypeStr=Inherit: Inherit via back propagation  NCopyOutMin=[]  NCopyOutMax=[]  IntegratorContinuousStateAttributes=''  IntegratorStateMustResolveToSignalObject=off  IntegratorRTWStateStorageClass=Auto  FilterContinuousStateAttributes=''  FilterStateMustResolveToSignalObject=off  FilterRTWStateStorageClass=Auto  ParallelPVariant=ExternalParameters  IdealPVariant=Disabled  IVariant=ExternalParameters  DVariant=ExternalParameters  IntegratorVariant=Continuous  SatVariant=Disabled  AWVariant=Passthrough  PCopyVariant=Disabled  TRVariant=Disabled  FdbkBlocksVariant=Forward  IdealPFdbkVariant=Disabled  SatFdbkVariant=Disabled  DerivativeFilterVariant=ContFilter  NVariant=ExternalParameters  NCopyVariant=Disabled  FilterICVariant=InternalICsFilter  IntegratorICVariant=InternalICs  ExternalResetVariant=Disabled  TRSumVariant=Passthrough  SumFdbkVariant=Disabled  SumVariant=Sum_PID  TsampFilterVariant=InternalTs  TsampNgainVariant=Passthrough  TsampIntegralVariant=Disabled_SignalSpec  ExternalSaturationOutDataTypeStr=Inherit: Same as second input  DerivativeSourceVariant=ErrorSignal  PreIntVariant=InternalPreInt
  Varying State Space : Subsystem  mask(Varying State Space){InitialConditionSource=internal, InitialCondition=0, xNames='', OutputX=on, OutputDX=on, Feedthrough=on, InputX0=off, InputDX0=off, InputU0=off, InputY0=off}
      mask prompts: InitialConditionSource "Simulink:blkprm_prompts:IntegratorInitCondSrc"; InitialCondition "Simulink:blkprm_prompts:IntegratorInitCond"; xNames "Control:simulink:VaryingSSLabel2"; OutputX "Control:simulink:VaryingSSLabel3"; OutputDX "Control:simulink:VaryingSSLabel4"; Feedthrough "Control:simulink:VaryingSSLabel6"; InputX0 "Control:simulink:VaryingSSLabel10"; InputDX0 "Control:simulink:VaryingSSLabel11"; InputU0 "Control:simulink:VaryingSSLabel12"; InputY0 "Control:simulink:VaryingSSLabel13"
      mask help: Control:simulink:VaryingSS1
      mask init:
      | if controllib.internal.blocks.safeMaskUpdate(gcb)
      |     Selection = struct('x',OutputX,'dx',OutputDX,'D',Feedthrough,...
      |         'x0',InputX0,'dx0',InputDX0,'u0',InputU0,'y0',InputY0,...
      |         'IC',strcmp(get_param(gcb,'InitialConditionSource'),'external'));
      |     if ~Selection.IC
      |         InitialCondition = InitialCondition(:);
      |     end
      |     controllib.internal.blocks.varying.varyingSS(gcb,Selection,0)
      | end
      mask Help: eval('helpview(''control'',''VaryingSSCT'');')
      mask TypeOptions InitialConditionSource: internal | external
      mask Callback InitialConditionSource: controllib.internal.blocks.varying.varyingSS_callback(gcb,'InitialConditionSource')
      mask DialogControl Container4 Prompt: Control:simulink:VaryingSSLabel7
      mask DialogControl InitialConditionSource Prompt: Initial condition source:
      mask DialogControl InitialCondition Prompt: Initial condition:
      mask DialogControl xNames Prompt: State names (e.g., 'position'):
      mask DialogControl OutputX Prompt: Output states
      mask DialogControl OutputDX Prompt: Output state derivatives
      mask DialogControl Feedthrough Prompt: Enable feedthrough D
      mask DialogControl Container5 Prompt: Control:simulink:VaryingSSLabel8
      mask DialogControl InputX0 Prompt: Enable state offsets x0
      mask DialogControl InputDX0 Prompt: Enable state derivative offsets dx0
      mask DialogControl InputU0 Prompt: Enable input offsets u0
      mask DialogControl InputY0 Prompt: Enable output offsets y0
      mask Display:
      | [eqx,eqy] = controllib.internal.blocks.varying.varyingSS_icon(true,Feedthrough,InputX0,InputDX0,InputU0,InputY0);
      | text(0.5,0.65,eqx,'horizontalAlignment', 'center','texmode','on')
      | text(0.5,0.35,eqy,'horizontalAlignment', 'center','texmode','on')
      | port_label('input', 1, 'u')
      | port_label('input', 2, 'A')
      | port_label('input', 3, 'B')
      | port_label('input', 4, 'C')
      | port_label('output', 1, 'y')
      | nout = 1;
      | if OutputX
      |    nout = nout+1;
      |    port_label('output', nout, 'x')
      | end
      | if OutputDX
      |    nout = nout+1;
      |    port_label('output', nout, 'dx')
      | end
      | nin = 4;
      | if Feedthrough
      |    nin = nin+1;
      |    port_label('input', nin, 'D')
      | end
      | if InputDX0
      |    nin = nin+1;
      |    port_label('input', nin, 'dx0')
      | end
      | if InputX0
      |    nin = nin+1;
      |    port_label('input', nin, 'x0')
      | end
      | if InputU0
      |    nin = nin+1;
      |    port_label('input', nin, 'u0')
      | end
      | if InputY0
      |    nin = nin+1;
      |    port_label('input', nin, 'y0')
      | end
      | if strcmp(get_param(gcb,'InitialConditionSource'),'external')
      |    nin = nin+1;
      |    port_label('input', nin, 'IC')
      | end
  Varying Transfer Function : Subsystem  mask(Varying Transfer Function){N=1, Feedthrough=on}
      mask prompts: N "Control:simulink:VaryingTFLabel1"; Feedthrough "Control:simulink:VaryingSSLabel6"
      mask help: Control:simulink:VaryingTF1
      mask init:
      | if N~=round(N)
      |    hCB = get_param(gcb,'handle');
      |    DAStudio.slerror('Control:simulink:InvalidOrder',hCB)
      | end
      | Ts = 0;
      | SimStatus = get_param(bdroot,'SimulationStatus');
      | if any(strcmp(SimStatus,{'initializing','updating','stopped'}))
      |    controllib.internal.blocks.varying.varyingTF(gcb,N,Ts,Feedthrough)
      | end
      mask Help: eval('helpview(''control'',''VaryingTFCT'');')
      mask DialogControl N Prompt: Transfer function order:
      mask DialogControl Feedthrough Prompt: Enable feedthrough D
      mask Display:
      | port_label('input',3,'a1');
      | port_label('input',2,'b0');
      | port_label('input',4,'b1');
      | plot([0.325 0.675],[0.5 0.5])
      | text(0.5, 0.7, 'b_0 + b_1 s^{-1}' ,...
      |         'horizontalAlignment', 'center','texmode','on')
      | text(0.5, 0.3, '1 + a_1 s^{-1}' ,...
      |         'horizontalAlignment', 'center','texmode','on')
